simulink model "full_system"  (R2023b)
settings: Solver=VariableStepAuto  StartTime=0.0  StopTime=Tend  RelTol=1e-3
settings Model: Creator=GLORIA  LastModifiedBy=joseg
settings OptimizationCC: ReuseModelBlockBuffer=off

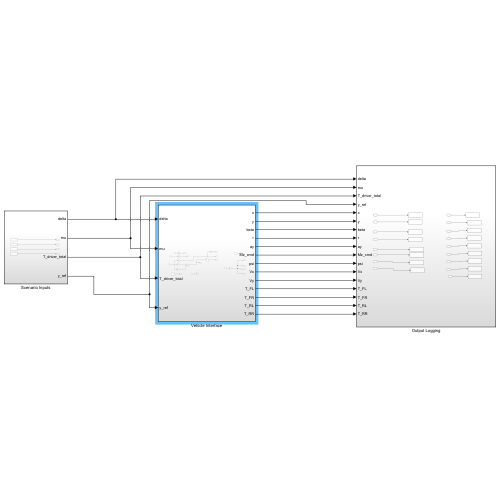
[thumbnail: Simulink's stored preview of the top-level diagram]
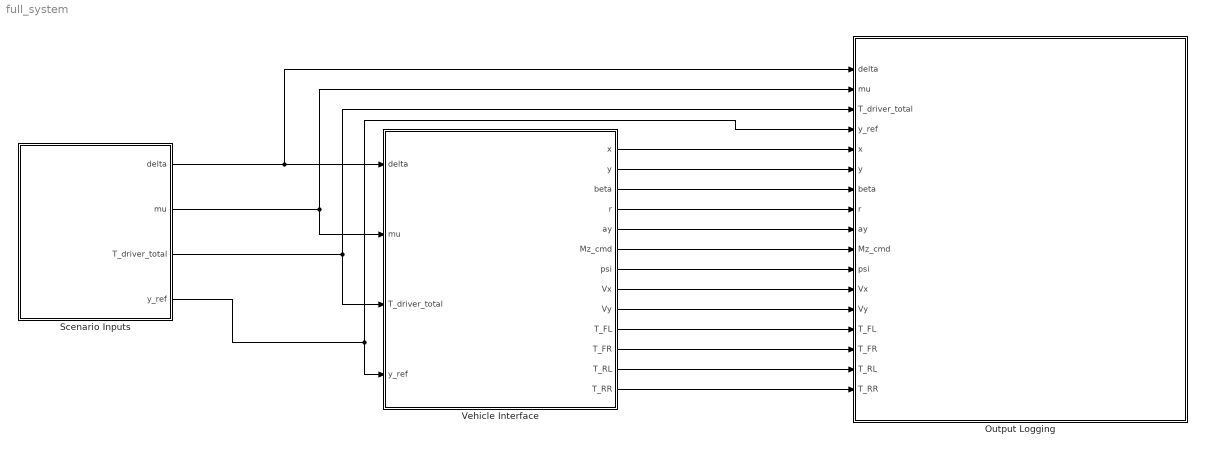
== system full_system ==
  Output Logging : Subsystem
  Scenario Inputs : Subsystem
  Vehicle Interface : Subsystem
  wires:
  Scenario Inputs/1(delta) -> Vehicle Interface/1(delta), Output Logging/1(delta)
  Scenario Inputs/2(mu) -> Output Logging/2(mu), Vehicle Interface/2(mu)
  Scenario Inputs/4(y_ref) -> Output Logging/4(y_ref), Vehicle Interface/4(y_ref)
  Vehicle Interface/1(x) -> Output Logging/5(x)
  Vehicle Interface/2(y) -> Output Logging/6(y)
  Vehicle Interface/3(beta) -> Output Logging/7(beta)
  Vehicle Interface/4(r) -> Output Logging/8(r)
  Vehicle Interface/5(ay) -> Output Logging/9(ay)
  Vehicle Interface/6(Mz_cmd) -> Output Logging/10(Mz_cmd)
  Vehicle Interface/7(psi) -> Output Logging/11(psi)
  Vehicle Interface/8(Vx) -> Output Logging/12(Vx)
  Vehicle Interface/9(Vy) -> Output Logging/13(Vy)
  Vehicle Interface/10(T_FL) -> Output Logging/14(T_FL)
  Vehicle Interface/11(T_FR) -> Output Logging/15(T_FR)
  Vehicle Interface/12(T_RL) -> Output Logging/16(T_RL)
  Vehicle Interface/13(T_RR) -> Output Logging/17(T_RR)
  Scenario Inputs/3(T_driver_total) -> Output Logging/3(T_driver_total), Vehicle Interface/3(T_driver_total)

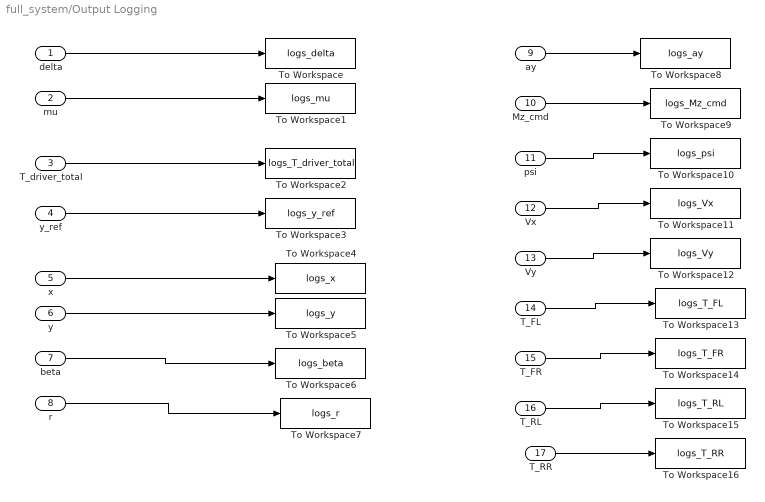
== system full_system/Output Logging ==
  delta : Inport
  mu : Inport  Port=2
  T_driver_total : Inport  Port=3
  y_ref : Inport  Port=4
  x : Inport  Port=5
  y : Inport  Port=6
  beta : Inport  Port=7
  r : Inport  Port=8
  ay : Inport  Port=9
  Mz_cmd : Inport  Port=10
  psi : Inport  Port=11
  Vx : Inport  Port=12
  Vy : Inport  Port=13
  T_FL : Inport  Port=14
  T_FR : Inport  Port=15
  T_RL : Inport  Port=16
  T_RR : Inport  Port=17
  To Workspace : ToWorkspace  VariableName=logs_delta  SaveFormat=Timeseries  SampleTime=-1
  To Workspace1 : ToWorkspace  VariableName=logs_mu  SaveFormat=Timeseries  SampleTime=-1
  To Workspace10 : ToWorkspace  VariableName=logs_psi  SaveFormat=Timeseries  SampleTime=-1
  To Workspace11 : ToWorkspace  VariableName=logs_Vx  SaveFormat=Timeseries  SampleTime=-1
  To Workspace12 : ToWorkspace  VariableName=logs_Vy  SaveFormat=Timeseries  SampleTime=-1
  To Workspace13 : ToWorkspace  VariableName=logs_T_FL  SaveFormat=Timeseries  SampleTime=-1
  To Workspace14 : ToWorkspace  VariableName=logs_T_FR  SaveFormat=Timeseries  SampleTime=-1
  To Workspace15 : ToWorkspace  VariableName=logs_T_RL  SaveFormat=Timeseries  SampleTime=-1
  To Workspace16 : ToWorkspace  VariableName=logs_T_RR  SaveFormat=Timeseries  SampleTime=-1
  To Workspace2 : ToWorkspace  VariableName=logs_T_driver_total  SaveFormat=Timeseries  SampleTime=-1
  To Workspace3 : ToWorkspace  VariableName=logs_y_ref  SaveFormat=Timeseries  SampleTime=-1
  To Workspace4 : ToWorkspace  VariableName=logs_x  SaveFormat=Timeseries  SampleTime=-1
  To Workspace5 : ToWorkspace  VariableName=logs_y  SaveFormat=Timeseries  SampleTime=-1
  To Workspace6 : ToWorkspace  VariableName=logs_beta  SaveFormat=Timeseries  SampleTime=-1
  To Workspace7 : ToWorkspace  VariableName=logs_r  SaveFormat=Timeseries  SampleTime=-1
  To Workspace8 : ToWorkspace  VariableName=logs_ay  SaveFormat=Timeseries  SampleTime=-1
  To Workspace9 : ToWorkspace  VariableName=logs_Mz_cmd  SaveFormat=Timeseries  SampleTime=-1
  wires:
  delta/1 -> To Workspace/1
  mu/1 -> To Workspace1/1
  T_driver_total/1 -> To Workspace2/1
  y_ref/1 -> To Workspace3/1
  x/1 -> To Workspace4/1
  y/1 -> To Workspace5/1
  beta/1 -> To Workspace6/1
  r/1 -> To Workspace7/1
  ay/1 -> To Workspace8/1
  Mz_cmd/1 -> To Workspace9/1
  psi/1 -> To Workspace10/1
  Vx/1 -> To Workspace11/1
  Vy/1 -> To Workspace12/1
  T_FL/1 -> To Workspace13/1
  T_FR/1 -> To Workspace14/1
  T_RL/1 -> To Workspace15/1
  T_RR/1 -> To Workspace16/1

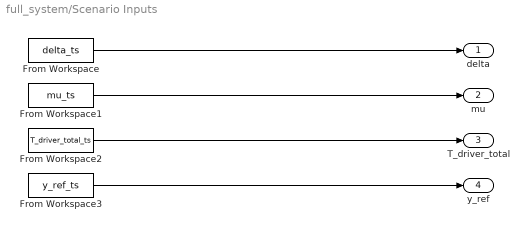
== system full_system/Scenario Inputs ==
  From Workspace : FromWorkspace  VariableName=delta_ts
  From Workspace1 : FromWorkspace  VariableName=mu_ts
  From Workspace2 : FromWorkspace  VariableName=T_driver_total_ts
  From Workspace3 : FromWorkspace  VariableName=y_ref_ts
  delta : Outport
  mu : Outport  Port=2
  T_driver_total : Outport  Port=3
  y_ref : Outport  Port=4
  wires:
  From Workspace/1 -> delta/1
  From Workspace1/1 -> mu/1
  From Workspace2/1 -> T_driver_total/1
  From Workspace3/1 -> y_ref/1

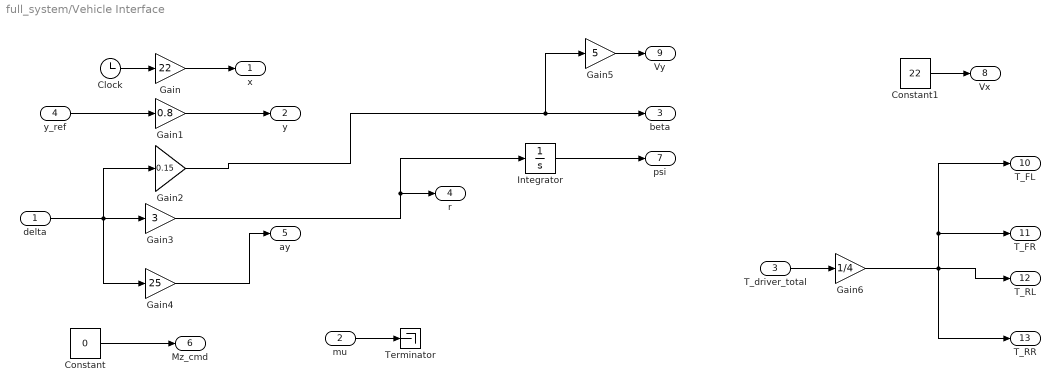
== system full_system/Vehicle Interface ==
  delta : Inport
  mu : Inport  Port=2
  T_driver_total : Inport  Port=3
  y_ref : Inport  Port=4
  Clock : Clock
  Constant : Constant  Value=0
  Constant1 : Constant  Value=22
  Gain : Gain  Gain=22
  Gain1 : Gain  Gain=0.8
  Gain2 : Gain  Gain=0.15
  Gain3 : Gain  Gain=3
  Gain4 : Gain  Gain=25
  Gain5 : Gain  Gain=5
  Gain6 : Gain  Gain=1/4
  Integrator : Integrator
  Terminator : Terminator
  x : Outport
  y : Outport  Port=2
  beta : Outport  Port=3
  r : Outport  Port=4
  ay : Outport  Port=5
  Mz_cmd : Outport  Port=6
  psi : Outport  Port=7
  Vx : Outport  Port=8
  Vy : Outport  Port=9
  T_FL : Outport  Port=10
  T_FR : Outport  Port=11
  T_RL : Outport  Port=12
  T_RR : Outport  Port=13
  wires:
  Clock/1 -> Gain/1
  Gain/1 -> x/1
  y_ref/1 -> Gain1/1
  Gain1/1 -> y/1
  Gain2/1 -> Gain5/1, beta/1
  delta/1 -> Gain4/1, Gain3/1, Gain2/1
  Gain3/1 -> Integrator/1, r/1
  Gain4/1 -> ay/1
  Constant/1 -> Mz_cmd/1
  Integrator/1 -> psi/1
  Constant1/1 -> Vx/1
  Gain5/1 -> Vy/1
  Gain6/1 -> T_RR/1, T_RL/1, T_FL/1, T_FR/1
  T_driver_total/1 -> Gain6/1
  mu/1 -> Terminator/1
